simulink model "aeb_model"  (R2025b)
settings: Solver=FixedStepDiscrete  StartTime=0.0  StopTime=0  FixedStep=1  RelTol=1e-3
settings Model: Creator=user  LastModifiedBy=user

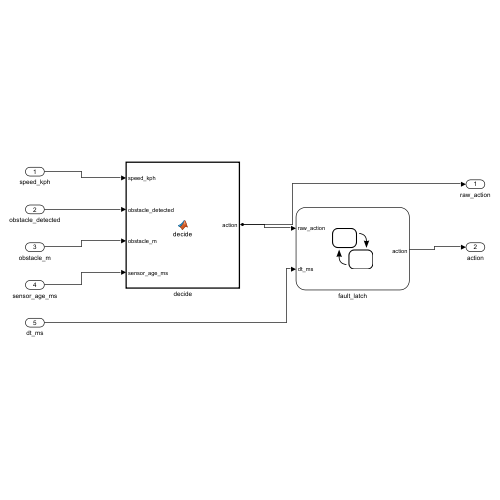
[thumbnail: Simulink's stored preview of the top-level diagram]
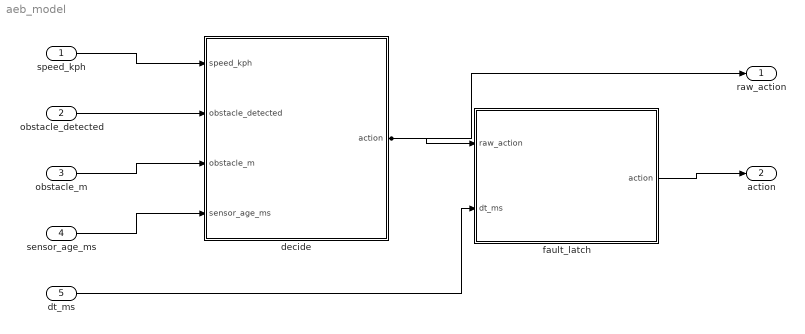
== system aeb_model ==
  speed_kph : Inport  OutDataTypeStr=double  SampleTime=1  Interpolate=off
  obstacle_detected : Inport  Port=2  OutDataTypeStr=double  SampleTime=1  Interpolate=off
  obstacle_m : Inport  Port=3  OutDataTypeStr=double  SampleTime=1  Interpolate=off
  sensor_age_ms : Inport  Port=4  OutDataTypeStr=double  SampleTime=1  Interpolate=off
  dt_ms : Inport  Port=5  OutDataTypeStr=double  SampleTime=1  Interpolate=off
  decide : MATLAB Function  TreatAsAtomicUnit=on
  fault_latch : Stateflow chart  TreatAsAtomicUnit=on
  raw_action : Outport
  action : Outport  Port=2
  wires:
  speed_kph/1 -> decide/1(speed_kph)
  obstacle_detected/1 -> decide/2(obstacle_detected)
  obstacle_m/1 -> decide/3(obstacle_m)
  sensor_age_ms/1 -> decide/4(sensor_age_ms)
  decide/1(action) -> raw_action/1, fault_latch/1(raw_action)
  dt_ms/1 -> fault_latch/2(dt_ms)
  fault_latch/1(action) -> action/1

== matlab function aeb_model/decide ==
  data: speed_kph input; action output; obstacle_detected input; obstacle_m input; sensor_age_ms input
function action = decide(speed_kph, obstacle_detected, obstacle_m, sensor_age_ms)
% Stateless AEB-lite decision. 0 NO_ACTION, 1 BRAKE, 2 FAULT.
SPEED_MIN = 0.0;
SPEED_MAX = 250.0;
BRAKE_SPEED_KPH = 30.0;
DETECT_RANGE_M = 20.0;
SENSOR_TIMEOUT_MS = 200;

if ~(speed_kph >= SPEED_MIN && speed_kph <= SPEED_MAX)
    action = 2;
elseif sensor_age_ms >= SENSOR_TIMEOUT_MS
    action = 2;
elseif speed_kph >= BRAKE_SPEED_KPH && obstacle_detected ~= 0 && obstacle_m <= DETECT_RANGE_M
    action = 1;
else
    action = 0;
end

== stateflow chart aeb_model/fault_latch ==
  settings: executeAtInitialization=1
  state NORMAL
    du: action = raw_action;
  state FAULT_LATCHED
    du:
    if raw_action == FAULT
    healthy_ms = 0;
    else
    healthy_ms = healthy_ms + dt_ms;
    end
    action = FAULT;
  (default) -> NORMAL
  FAULT_LATCHED -> NORMAL : [raw_action ~= FAULT && healthy_ms + dt_ms >= RECOVERY_MS]
      | {healthy_ms = 0; action = raw_action;}
  NORMAL -> FAULT_LATCHED : [raw_action == FAULT]
      | {healthy_ms = 0; action = FAULT;}
  data: raw_action input; dt_ms input; action output =0; healthy_ms local =0; FAULT constant double =2; RECOVERY_MS constant double =1000
